simulink model "mpc_period_with_r_and_d_simulink"  (R2015a)
settings: Solver=ode45  SolverMode=SingleTasking  StartTime=0.0  StopTime=simu.time  RelTol=1e-3
values from neighbouring files (symbols this model uses):
  plant = tf([3], [tau 1])    [mpc_period_exp.m]
undefined symbols (not defined in the file or in its folder): mpc_param, simu
libraries: mpclib x1
settings Model: CovSFcnEnable=off  ExtModeTrigMode=oneshot  ExtModeArmWhenConnect=off  Creator=The MathWorks Inc.  LastModifiedBy=Xiaotian
settings DataIOCC: LimitDataPoints=off  SaveOutput=off  SignalLogging=off  DSMLogging=off  SaveTime=off  SignalLoggingName=sigsOut
settings OptimizationCC: BooleanDataType=off  ExpressionDepthLimit=2147483647  InitFltsAndDblsToZero=on
settings DebuggingCC: SaveWithParameterizedLinksMsg=none  UnderspecifiedInitializationDetection=Classic  MergeDetectMultiDrivingBlocksExec=none  SignalResolutionControl=TryResolveAllWithWarning  MultiTaskDSMMsg=warning  MultiTaskCondExecSysMsg=none  IntegerOverflowMsg=none  FcnCallInpInsideContextMsg=UseLocalSettings  StateNameClashWarn=warning  IntegerSaturationMsg=none
settings HardwareCC: TargetUnknown=on
settings GRTTargetCC: TargetFcnLib=ansi_tfl_tmw.mat  CombineOutputUpdateFcns=off  GRTInterface=on

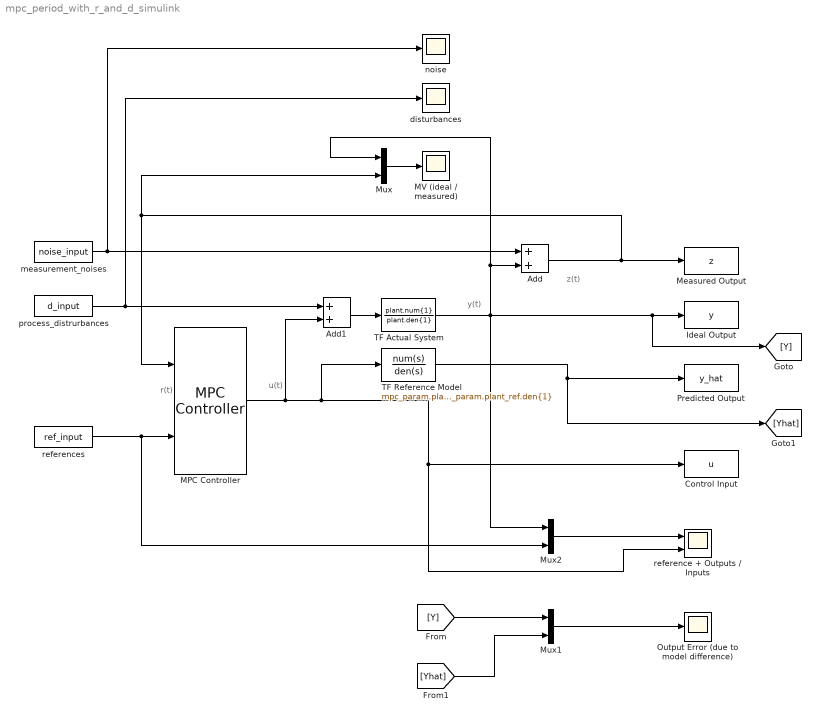
== system mpc_period_with_r_and_d_simulink ==
  note: r(t)
  note: u(t)
  note: y(t)
  note: z(t)
  Add : Sum
  Add1 : Sum
  Control Input : ToWorkspace  VariableName=u  SampleTime=simu.samlping_time
      settings: MaxDataPoints=Inf
  Ideal Output : ToWorkspace  VariableName=y  SampleTime=simu.samlping_time
      settings: MaxDataPoints=Inf
  MPC Controller : mpclib/MPC Controller  mpcobj=mpcobj  x0=[]  is_multiple=0  enable_value=0  n_mv=1  n_mo=1  n_md=0  n_ts=0.01  is_designfromscratch=0  return_u0=off  ref_from_ws=off  ref_signal_name=[]  ref_preview=on  md_from_ws=off  md_signal_name=[]  md_preview=on  from_project=off  project_file=MPCtask.mat  md_inport=off  mv_inport=off  cost_outport=off  return_sequence=off  return_qpstatus=off  return_state=off  state_inport=off  lims_inport=off  ywt_inport=off  uwt_inport=off  duwt_inport=off  rhoeps_inport=off  uref_inport=off  BlockDataType=double  SampleTimeInherited=off  switch_inport=off
  MV (ideal / measured) : Scope
      settings: TimeRange=10  YMin=-1.5  YMax=1.75  DataFormat=Structure
  Measured Output : ToWorkspace  VariableName=z  SampleTime=simu.samlping_time
      settings: MaxDataPoints=Inf
  Mux : Mux  Inputs=2
  Mux1 : Mux  Inputs=2
  Mux2 : Mux  Inputs=2
  Output Error (due to model difference) : Scope
      settings: TimeRange=10  YMin=-29.95  YMax=-29.6  SaveName=ScopeData2  DataFormat=Structure  SampleInput=on  SampleTime=simu.samlping_time
  Predicted Output : ToWorkspace  VariableName=y_hat  SampleTime=simu.samlping_time
      settings: MaxDataPoints=Inf
  TF Actual System : TransferFcn  Numerator=plant.num{1}  Denominator=plant.den{1}
  TF Reference Model : TransferFcn  Numerator=mpc_param.plant_ref.num{1}  Denominator=mpc_param.plant_ref.den{1}
  disturbances : Scope
      settings: TimeRange=10  YMin=-29.95  YMax=-29.6  SaveName=ScopeData4  DataFormat=Structure  SampleInput=on  SampleTime=simu.samlping_time
  measurement_noises : FromWorkspace  VariableName=noise_input  SampleTime=0
  noise : Scope
      settings: TimeRange=10  YMin=-29.95  YMax=-29.6  SaveName=ScopeData3  DataFormat=Structure  SampleInput=on  SampleTime=simu.samlping_time
  process_distrurbances : FromWorkspace  VariableName=d_input  SampleTime=0
  reference + Outputs / Inputs : Scope  NumInputPorts=2
      settings: TimeRange=10  YMin=-0.5~-1  YMax=4.5~1.5  DataFormat=Structure  SampleInput=on  SampleTime=simu.samlping_time
  references : FromWorkspace  VariableName=ref_input  SampleTime=0
  wires:
  MPC Controller/1 -> Add1/2, reference + Outputs / Inputs/2, Control Input/1, TF Reference Model/1
  TF Actual System/1 -> Mux2/1, Mux/1, Add/2, [Y], Ideal Output/1
  references/1 -> Mux2/2, MPC Controller/2
  Add/1 -> Measured Output/1, MPC Controller/1, Mux/2
  measurement_noises/1 -> noise/1, Add/1
  Add1/1 -> TF Actual System/1
  process_distrurbances/1 -> disturbances/1, Add1/1
  Mux/1 -> MV (ideal / measured)/1
  TF Reference Model/1 -> [Yhat], Predicted Output/1
  Mux1/1 -> Output Error (due to model difference)/1
  [Y] -> Mux1/1
  [Yhat] -> Mux1/2
  Mux2/1 -> reference + Outputs / Inputs/1
